simulink library "project2lib"  (R2017b)
settings: Solver=VariableStepAuto  StartTime=0.0  StopTime=10.0  RelTol=1e-3
libraries: untitled x1, realtime_pacer_lib x1
settings Model: Creator=ibrahim  LastModifiedBy=minh
settings CodeAppCC: StateflowObjectComments=on

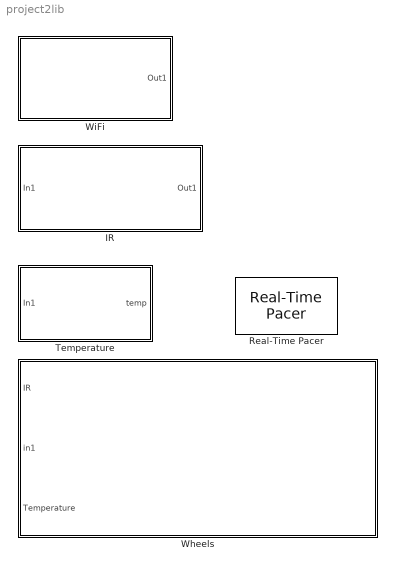
== system project2lib ==
  "IR " : Subsystem
  Real-Time Pacer : realtime_pacer_lib/Real-Time Pacer  simTimePerRealTime=.5
  Temperature : Subsystem
  Wheels : Subsystem
  WiFi : Subsystem

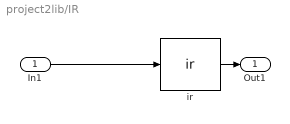
== system project2lib/IR  ==
  In1 : Inport
  ir : untitled/Subsystem1/ir
  Out1 : Outport
  wires:
  ir/1 -> Out1/1
  In1/1 -> ir/1

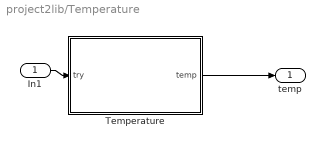
== system project2lib/Temperature ==
  In1 : Inport
  Temperature : Stateflow chart  TreatAsAtomicUnit=on
  temp : Outport
  wires:
  In1/1 -> Temperature/1(try)
  Temperature/1(temp) -> temp/1

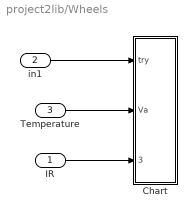
== system project2lib/Wheels ==
  IR : Inport
  in1 : Inport  Port=2
  Temperature : Inport  Port=3
  Chart : Stateflow chart  TreatAsAtomicUnit=on
  wires:
  in1/1 -> Chart/1(try)
  Temperature/1 -> Chart/2(Va)
  IR/1 -> Chart/3(input1)

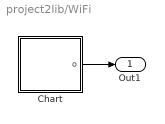
== system project2lib/WiFi ==
  Chart : Stateflow chart  AncestorBlock=untitled/Init/Chart  TreatAsAtomicUnit=on
  Out1 : Outport
  wires:
  Chart/1(o) -> Out1/1

== stateflow chart project2lib/Temperature/Temperature ==
  state temp
    en,du:
    temp=T;
  (default) -> temp
  data: y function_output; try input; temp output
  function y= T:
    | function y= T
    | persistent so
    | y=1;
    | coder.extrinsic('evalin');
    | coder.extrinsic('get');
    | 
    | so = evalin('base','objWs');
    | 
    | temp=0;  
    | coder.extrinsic('TemperatureRoomba');
    | temp=TemperatureRoomba(so);
    | 
    | y=temp;

== stateflow chart project2lib/WiFi/Chart ==
  state fist
    en,du:
    tcpInit;
    o=1;
  (default) -> fist
  data: o output
  function tcpInit:
    | function tcpInit
    | coder.extrinsic('RoombaInitfanny');
    | coder.extrinsic('assignin');
    | persistent obj
    | if isempty(obj)
    |     obj=RoombaInitfanny('10.0.0.1','full');
    |     assignin('base','objWs',obj);
    | end

== stateflow chart project2lib/Wheels/Chart ==
  state on1
    state off
      en,du:
      Wheels(0,0);
    state on
      state Reverse
        entry:
        Wheels(-.1,-0.1);
      state Straiforward
        entry,du:
        Wheels(0.05,0.05);
      state Rightturn3
        entry,du:
        Wheels(-0.2,0.2);
      state leftturn3
        entry,du:
        Wheels(0.2,-0.2);
      state Leftturn3
        entry,du:
        Wheels(0.3,-0.2);
      state Rightturn2
        entry,du:
        Wheels(-0.2,0.3);
      state Leftturn2
        entry,du:
        Wheels(.2,              -0.1);
      state Rightturn1
        entry,du:
        Wheels(-0.1,.2);
      (default) -> Reverse
      Reverse -> Straiforward : after(1,sec)
      Straiforward -> Rightturn1 [order 1] : [input1(1)>0]
      Rightturn1 -> Straiforward : [input1(1)<1]
      Straiforward -> Rightturn2 [order 2] : [input1(2)>0]
      Rightturn2 -> Straiforward : [input1(2)<1]
      Straiforward -> Rightturn3 [order 3] : [input1(3)>0]
      Rightturn3 -> Straiforward : [input1(3)<1]
      Straiforward -> leftturn3 [order 4] : [input1(4)>0]
      leftturn3 -> Straiforward : [input1(4)<1]
      Straiforward -> Leftturn3 [order 5] : [input1(5)>0]
      Leftturn3 -> Straiforward : [input1(5)<1]
      Straiforward -> Leftturn2 [order 6] : [input1(6)>0]
      Leftturn2 -> Straiforward : [input1(6)<1]
    (default) -> off
    off -> on : [Va<80]
    on -> off : [Va>=80]
  (default) -> on1
  data: u1 function_input; u2 function_input; try input; Va input; input1 input
  function Wheels(u1,u2):
    | function Wheels(u1,u2)
    | persistent so
    | coder.extrinsic('evalin');
    | coder.extrinsic('get');
    | so = evalin('base','objWs');
    | coder.extrinsic('SetWheelVelRoomba');
    | SetWheelVelRoomba(so,u1 , u2);
